simulink model "lab1_RobustStateSpaceController"  (R2020b)
settings: Solver=VariableStepAuto  StartTime=0.0  StopTime=3  RelTol=1e-3
undefined symbols (not defined in the file): D_w, degs2rpm, K, K_I, N_r, N_w, rpm2rads, sens, stepAmplitude
settings Model: Creator=Musta  LastModifiedBy=Musta

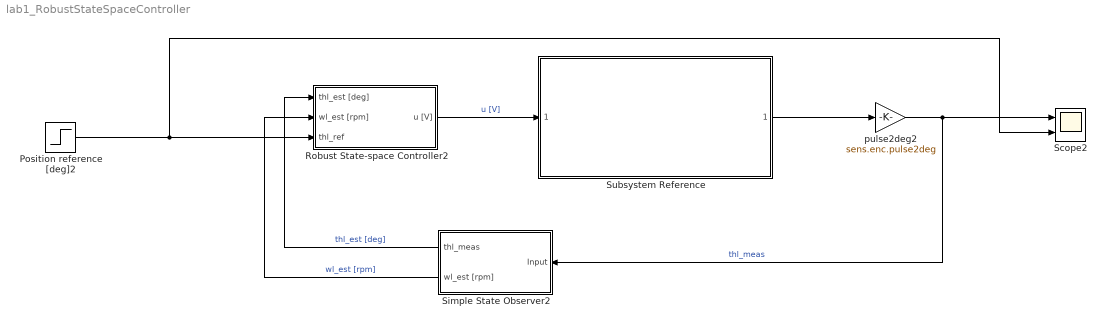
== system lab1_RobustStateSpaceController ==
  Position reference [deg]2 : Step  Time=0  After=stepAmplitude  SampleTime=0
  Robust State-space Controller2 : Subsystem
  Scope2 : Scope  NumInputPorts=2
  Simple State Observer2 : Subsystem
  Subsystem Reference : Subsystem  ReferencedSubsystem=plant_Model
  pulse2deg2 : Gain  Gain=sens.enc.pulse2deg
  wires:
  Position reference [deg]2/1 -> Scope2/2, Robust State-space Controller2/3(thl_ref)
  pulse2deg2/1 -> Scope2/1, Simple State Observer2/1(Input)  "thl_meas"
  Robust State-space Controller2/1(u [V]) -> Subsystem Reference/1  "u [V]"
  Simple State Observer2/2(wl_est [rpm]) -> Robust State-space Controller2/2(wl_est [rpm])  "wl_est [rpm]"
  Subsystem Reference/1 -> pulse2deg2/1
  Simple State Observer2/1(thl_meas) -> Robust State-space Controller2/1(thl_est [deg])  "thl_est [deg]"

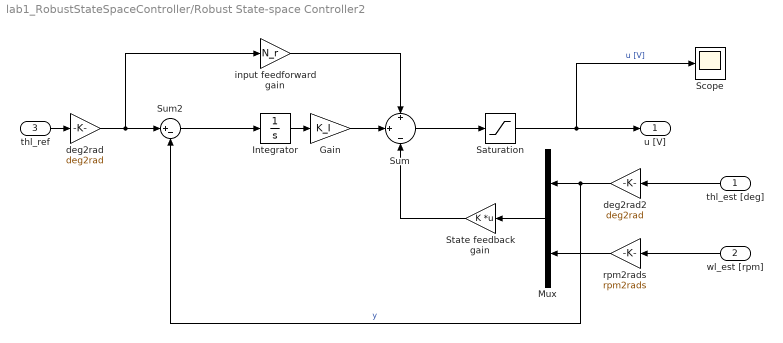
== system lab1_RobustStateSpaceController/Robust State-space Controller2 ==
  thl_est [deg] : Inport
  wl_est [rpm] : Inport  Port=2
  thl_ref : Inport  Port=3
  Gain : Gain  Gain=K_I
  Integrator : Integrator
  Mux : Mux  Inputs=2
  Saturation : Saturate  UpperLimit=10  LowerLimit=-10
  Scope : Scope
  State feedback gain : Gain  Gain=K  Multiplication=Matrix(K*u)
  Sum : Sum  Inputs=+|+|-
  Sum2 : Sum  Inputs=|+-
  deg2rad : Gain  Gain=deg2rad
  deg2rad2 : Gain  Gain=deg2rad
  input feedforward gain : Gain  Gain=N_r
  rpm2rads : Gain  Gain=rpm2rads
  u [V] : Outport
  wires:
  input feedforward gain/1 -> Sum/1
  Mux/1 -> State feedback gain/1
  deg2rad/1 -> Sum2/1, input feedforward gain/1
  Saturation/1 -> u [V]/1, Scope/1  "u [V]"
  rpm2rads/1 -> Mux/2
  deg2rad2/1 -> Sum2/2, Mux/1  "y"
  Integrator/1 -> Gain/1
  Gain/1 -> Sum/2
  State feedback gain/1 -> Sum/3
  Sum/1 -> Saturation/1
  Sum2/1 -> Integrator/1
  thl_est [deg]/1 -> deg2rad2/1
  wl_est [rpm]/1 -> rpm2rads/1
  thl_ref/1 -> deg2rad/1

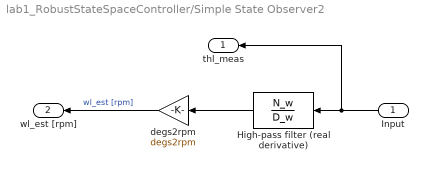
== system lab1_RobustStateSpaceController/Simple State Observer2 ==
  Input : Inport
  High-pass filter (real derivative) : TransferFcn  Numerator=N_w  Denominator=D_w
  degs2rpm : Gain  Gain=degs2rpm
  thl_meas : Outport
  wl_est [rpm] : Outport  Port=2
  wires:
  Input/1 -> thl_meas/1, High-pass filter (real derivative)/1
  High-pass filter (real derivative)/1 -> degs2rpm/1
  degs2rpm/1 -> wl_est [rpm]/1  "wl_est [rpm]"
